simulink model "Motore"  (R2023b)
settings: Solver=ode15s  StartTime=0.0  StopTime=7  MaxStep=1e-4  RelTol=1e-3
InitFcn:
  | %Parametri motore
  | 
  | Ra = 2.33;
  | La = 4e-3;
  | kv = 0.126; kt = kv;
  | Jtot = 7.77e-4;
  | 
  | B = 1.0051e-05;
  | 
  | % Costruzione fdt
  | 
  | P_el = tf(1,[La Ra]);
  | P_mec = tf(1,[Jtot B]);
libraries: cstblocks x2
settings Model: Creator=aniello  LastModifiedBy=aniello
settings ModelReferenceCC: ModelReferenceNumInstancesAllowed=Single

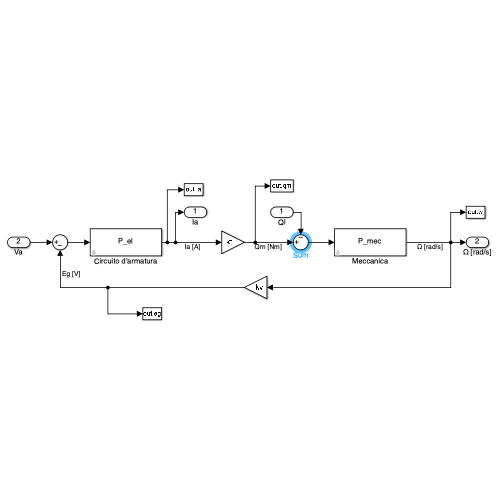
[thumbnail: Simulink's stored preview of the top-level diagram]
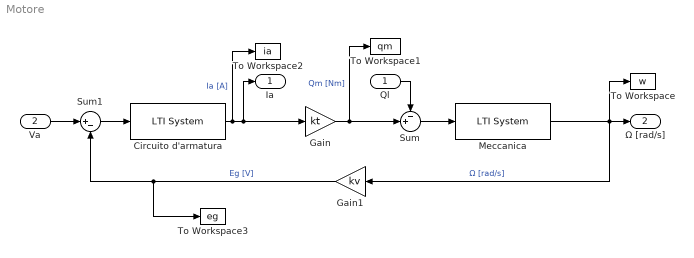
== system Motore ==
  Ql : Inport
  Va : Inport  Port=2
  Circuito d'armatura : cstblocks/LTI System  sys=P_el  IC=[]  PadeOrder=0
  Gain : Gain  Gain=kt
  Gain1 : Gain  Gain=kv
  Meccanica : cstblocks/LTI System  sys=P_mec  IC=[]  PadeOrder=0
  Sum : Sum  Inputs=-+|
  Sum1 : Sum  Inputs=|+-
  To Workspace : ToWorkspace  VariableName=w  SaveFormat=Timeseries  SampleTime=-1
  To Workspace1 : ToWorkspace  VariableName=qm  SaveFormat=Timeseries  SampleTime=-1
  To Workspace2 : ToWorkspace  VariableName=ia  SaveFormat=Timeseries  SampleTime=-1
  To Workspace3 : ToWorkspace  VariableName=eg  SaveFormat=Timeseries  SampleTime=-1
  Ia : Outport
  Ω [rad/s] : Outport  Port=2
  wires:
  Gain1/1 -> To Workspace3/1, Sum1/2  "Eg [V]"
  Gain/1 -> To Workspace1/1, Sum/2  "Qm [Nm]"
  Sum/1 -> Meccanica/1
  Sum1/1 -> Circuito d'armatura/1
  Circuito d'armatura/1 -> To Workspace2/1, Ia/1, Gain/1  "Ia [A]"
  Meccanica/1 -> Ω [rad/s]/1, Gain1/1, To Workspace/1  "Ω [rad/s]"
  Ql/1 -> Sum/1
  Va/1 -> Sum1/1
